simulink model "COV_sim_LQ_nonlin"  (R2023a)
settings: Solver=VariableStepAuto  StartTime=0.0  StopTime=tf  RelTol=1e-10
values from neighbouring files (symbols this model uses):
  alpha = 1/2.5    (= 0.4)    [COV_init_LQ_nonlin.m]
  c1 = feedback_pars(1)    [COV_init_LQ_nonlin.m]
  c2 = feedback_pars(2)    [COV_init_LQ_nonlin.m]
  c3 = feedback_pars(3)    [COV_init_LQ_nonlin.m]
  delta = 0.75    [COV_init_LQ_nonlin.m]
  dt = 0.1    [COV_init_LQ_nonlin.m]    (also in SLPIAHRD_transition.m = 0.02)
  ekf_sample_time = 0.02    [COV_init_LQ_nonlin.m]
  eta = 0.076    [COV_init_LQ_nonlin.m]
  h = 1/10    (= 0.1)    [COV_init_LQ_nonlin.m]    (also in mf_epid_ode_model_8comp.m = {})
  input_sample_time = 0.1    [COV_init_LQ_nonlin.m]
  k2 = 0.37    [COV_init_LQ_nonlin.m]
  k2_error = 1    [COV_init_LQ_nonlin.m]
  k3 = 0.1429    [COV_init_LQ_nonlin.m]
  k3_error = 1    [COV_init_LQ_nonlin.m]
  mu = 0.145    [COV_init_LQ_nonlin.m]
  N = numel(d_sim)-1    [Aggregator_B.m]    (also in Aggregator_C.m; COV_init_LQ_nonlin.m = 1; Main_MPC_Agent_v1.m = 168; Main_MPC_Agent_v2_Integral.m = P*Nr_Periods)
  p = 1/3    (= 0.333333333333)    [COV_init_LQ_nonlin.m]    (also in Main_MPC_Agent_v2_Integral.m = zeros(np,1); SLPIAHRD_transition.m = [1/2.5; 1/3; 1/3; 0.75; 0.6; 1/4; 1/4; 0.076; 1/10; 0.145])
  p_A = 1/4    (= 0.25)    [COV_init_LQ_nonlin.m]
  p_I = 1/4    (= 0.25)    [COV_init_LQ_nonlin.m]
  q = 0.6    [COV_init_LQ_nonlin.m]
  ref_sample_time = -1    [COV_init_LQ_nonlin.m]
  switchtime = 30    [COV_init_LQ_nonlin.m]
  u_max = k1    (= 0.5)    [COV_init_LQ_nonlin.m]
  u_min = 0    [COV_init_LQ_nonlin.m]
  x0 = [S0; L0; P0; A0; I0; R0; H0; D0]    [COV_init_LQ_nonlin.m]    (also in Main_MPC_Agent_v1.m = simx; Main_MPC_Agent_v2_Integral.m = simx; Main_MPC_Agent_v3.m = simx; Main_MPC_Agent_v5_Tp01.m = simx)
  z1_start = abs(x_ref(1, 2) - I0)    [COV_init_LQ_nonlin.m]
libraries: sharedTrackingLibrary x2
settings Model: PacingRate=0.001000  Creator=szeder  LastModifiedBy=ppolcz
settings SolverCC: ZeroCrossAlgorithm=Adaptive  AlgebraicLoopSolver=TrustRegion
settings OptimizationCC: ReuseModelBlockBuffer=off
settings DebuggingCC: UnconnectedInputMsg=warning  UnconnectedOutputMsg=warning  UnconnectedLineMsg=warning
settings ModelReferenceCC: EnableRefExpFcnMdlSchedulingChecks=on
settings RTWCC: DLArmComputeVersion=19.05

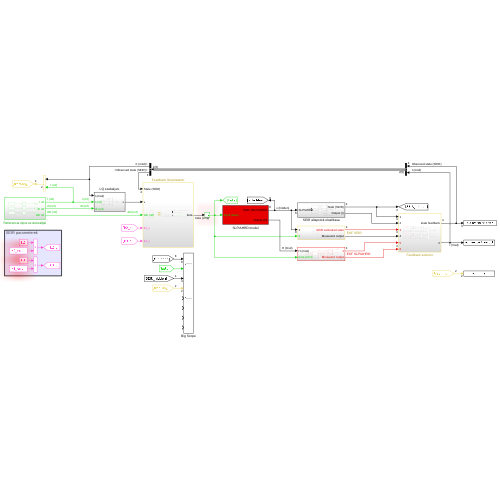
[thumbnail: Simulink's stored preview of the top-level diagram]
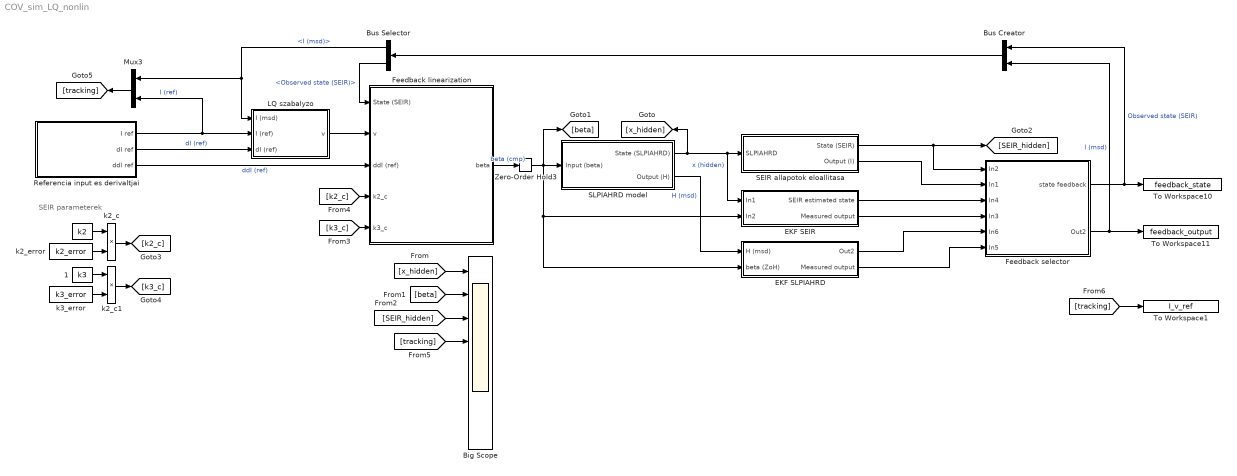
== system COV_sim_LQ_nonlin ==
  note: SEIR parameterek
  " " : Constant  Value=k2
  " 1" : Constant  Value=k3
  Big Scope : Scope  NumInputPorts=8
  Bus Creator : BusCreator  Inputs=2
  Bus Selector : BusSelector  OutputSignals=I (msd),Observed state (SEIR)
  EKF SEIR : Subsystem
  EKF SLPIAHRD : Subsystem
  Feedback linearization : Subsystem
  Feedback selector : Subsystem
  LQ szabalyzo : Subsystem
  Mux3 : Mux  Inputs=2
  Referencia input es derivaltjai : Subsystem
  SEIR allapotok eloallitasa : Subsystem
  SLPIAHRD model : Subsystem
  To Workspace1 : ToWorkspace  VariableName=I_v_ref  SaveFormat=Structure With Time  SampleTime=-1
  To Workspace10 : ToWorkspace  VariableName=feedback_state  SaveFormat=Timeseries  SampleTime=-1
  To Workspace11 : ToWorkspace  VariableName=feedback_output  SaveFormat=Timeseries  SampleTime=-1
  Zero-Order Hold3 : ZeroOrderHold  SampleTime=input_sample_time
  k2_c : Product
  k2_c1 : Product
  k2_error : Constant  Value=k2_error
  k3_error : Constant  Value=k3_error
  wires:
  Zero-Order Hold3/1 -> EKF SLPIAHRD/2(beta (ZoH)), EKF SEIR/2(In2), [beta], SLPIAHRD model/1(Input (beta))
  LQ szabalyzo/1(v) -> Feedback linearization/2(v)
  SLPIAHRD model/1(State (SLPIAHRD)) -> EKF SEIR/1(In1), SEIR allapotok eloallitasa/1(SLPIAHRD), [x_hidden]  "x (hidden)"
  SLPIAHRD model/2(Output (H)) -> EKF SLPIAHRD/1(H (msd))  "H (msd)"
  SEIR allapotok eloallitasa/1(State (SEIR)) -> [SEIR_hidden], Feedback selector/1(In2)
  Feedback selector/1(state feedback) -> To Workspace10/1, Bus Creator/1  "Observed state (SEIR)"
  Feedback selector/2(Out2) -> To Workspace11/1, Bus Creator/2  "I (msd)"
  SEIR allapotok eloallitasa/2(Output (I)) -> Feedback selector/2(In1)
  EKF SEIR/2(Measured output) -> Feedback selector/4(In3)
  EKF SEIR/1(SEIR estimated state) -> Feedback selector/3(In4)
  EKF SLPIAHRD/2(Measured output) -> Feedback selector/6(In5)
  EKF SLPIAHRD/1(Out2) -> Feedback selector/5(In6)
  Referencia input es derivaltjai/1(I ref) -> Mux3/2, LQ szabalyzo/2(I (ref))  "I (ref)"
  Referencia input es derivaltjai/2(dI ref) -> LQ szabalyzo/3(dI (ref))  "dI (ref)"
  Referencia input es derivaltjai/3(ddI ref) -> Feedback linearization/3(ddI (ref))  "ddI (ref)"
  [x_hidden] -> Big Scope/1
  [beta] -> Big Scope/2
  [SEIR_hidden] -> Big Scope/3
  " "/1 -> k2_c/1
  k2_error/1 -> k2_c/2
  [k2_c] -> Feedback linearization/4(k2_c)
  [k3_c] -> Feedback linearization/5(k3_c)
  k2_c/1 -> [k2_c]
  k2_c1/1 -> [k3_c]
  k3_error/1 -> k2_c1/2
  " 1"/1 -> k2_c1/1
  Mux3/1 -> [tracking]
  [tracking] -> Big Scope/4
  [tracking] -> To Workspace1/1
  Bus Creator/1 -> Bus Selector/1
  Bus Selector/1 -> Mux3/1, LQ szabalyzo/1(I (msd))  "<I (msd)>"
  Bus Selector/2 -> Feedback linearization/1(State (SEIR))  "<Observed state (SEIR)>"
  Feedback linearization/1(beta) -> Zero-Order Hold3/1  "beta (cmp)"

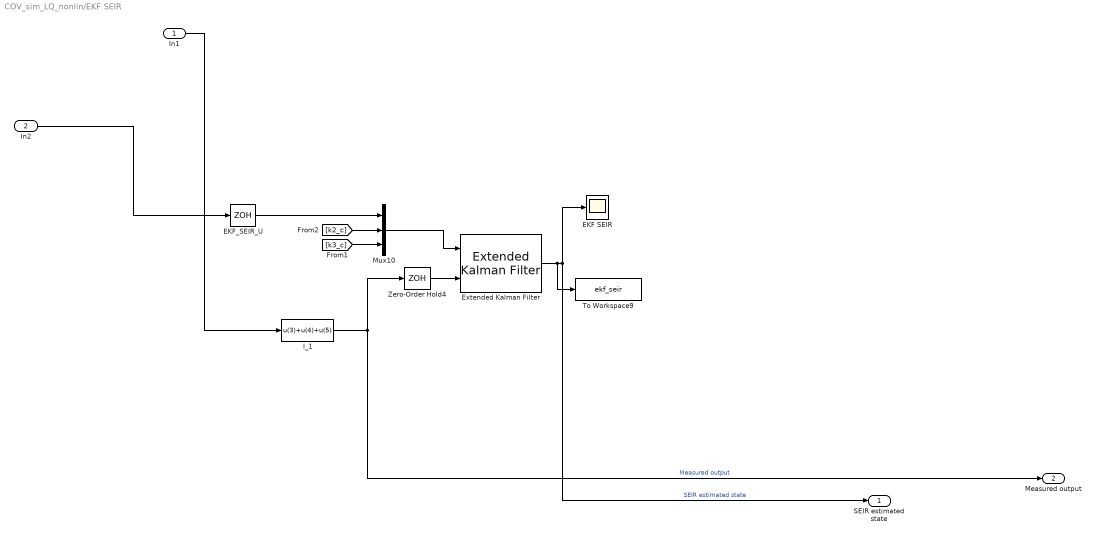
== system COV_sim_LQ_nonlin/EKF SEIR ==
  In1 : Inport
  In2 : Inport  Port=2
  EKF SEIR : Scope
  EKF_SEIR_U : ZeroOrderHold  SampleTime=ekf_sample_time
  Extended Kalman Filter : sharedTrackingLibrary/Extended Kalman Filter  StateTransitionFcn=SEIR_transition  HasStateTransitionJacobianFcn=off  HasAdditiveProcessNoise=Additive  ProcessNoise=ekf_seir_processcov  HasTimeVaryingProcessNoise=off  HasStateTransitionFcnExtraArgument=1  InitialState=ekf_seir_initialstate  InitialStateCovariance=ekf_seir_initcov  MeasurementFcn1=SEIR_measurement  HasMeasurementJacobianFcn1=off  HasMeasurementEnablePort1=off  HasAdditiveMeasurementNoise1=Additive  MeasurementNoise1=ekf_seir_measurecov  HasTimeVaryingMeasurementNoise1=off  HasMeasurementFcnExtraArgument1=0  HasMeasurementWrapping1=off  MeasurementFcn2=myMeasurementFcn  HasMeasurementJacobianFcn2=off  HasMeasurementEnablePort2=off  HasAdditiveMeasurementNoise2=Additive  MeasurementNoise2=1  HasTimeVaryingMeasurementNoise2=off  HasMeasurementFcnExtraArgument2=0  HasMeasurementWrapping2=off  MeasurementFcn3=myMeasurementFcn  HasMeasurementJacobianFcn3=off  HasMeasurementEnablePort3=off  HasAdditiveMeasurementNoise3=Additive  MeasurementNoise3=1  HasTimeVaryingMeasurementNoise3=off  HasMeasurementFcnExtraArgument3=0  HasMeasurementWrapping3=off  MeasurementFcn4=myMeasurementFcn  HasMeasurementJacobianFcn4=off  HasMeasurementEnablePort4=off  HasAdditiveMeasurementNoise4=Additive  MeasurementNoise4=1  HasTimeVaryingMeasurementNoise4=off  HasMeasurementFcnExtraArgument4=0  HasMeasurementWrapping4=off  MeasurementFcn5=myMeasurementFcn  HasMeasurementJacobianFcn5=off  HasMeasurementEnablePort5=off  HasAdditiveMeasurementNoise5=Additive  MeasurementNoise5=1  HasTimeVaryingMeasurementNoise5=off  HasMeasurementFcnExtraArgument5=0  HasMeasurementWrapping5=off  EnableMultirate=off  StateTransitionFcnSampleTime=1  MeasurementFcn1SampleTime=1  MeasurementFcn2SampleTime=1  MeasurementFcn3SampleTime=1  MeasurementFcn4SampleTime=1  MeasurementFcn5SampleTime=1  UseCurrentEstimator=on  OutputStateCovariance=off  DataType=double  SampleTime=ekf_sample_time  NumberOfMeasurements=1
  I_1 : MATLABFcn  MATLABFcn=u(3)+u(4)+u(5)  OutputDimensions=1  Output1D=off
  Mux10 : Mux  Inputs=3
  To Workspace9 : ToWorkspace  VariableName=ekf_seir  SaveFormat=Timeseries  SampleTime=-1
  Zero-Order Hold4 : ZeroOrderHold  SampleTime=ekf_sample_time
  SEIR estimated state : Outport
  Measured output : Outport  Port=2
  wires:
  EKF_SEIR_U/1 -> Mux10/1
  [k3_c] -> Mux10/3
  Zero-Order Hold4/1 -> Extended Kalman Filter/2
  In2/1 -> EKF_SEIR_U/1
  I_1/1 -> Measured output/1, Zero-Order Hold4/1  "Measured output"
  Mux10/1 -> Extended Kalman Filter/1
  Extended Kalman Filter/1 -> SEIR estimated state/1, EKF SEIR/1, To Workspace9/1  "SEIR estimated state"
  [k2_c] -> Mux10/2
  In1/1 -> I_1/1

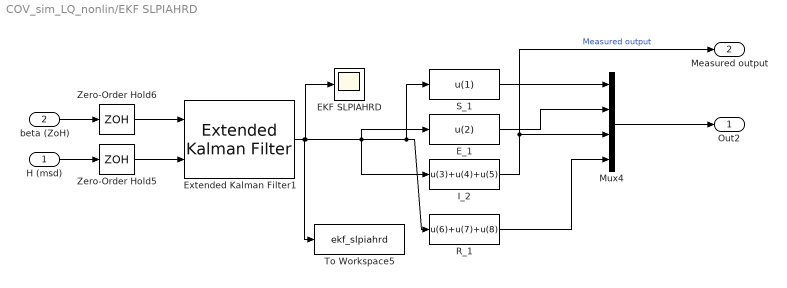
== system COV_sim_LQ_nonlin/EKF SLPIAHRD ==
  H (msd) : Inport
  beta (ZoH) : Inport  Port=2
  EKF SLPIAHRD : Scope
  E_1 : MATLABFcn  MATLABFcn=u(2)
  Extended Kalman Filter1 : sharedTrackingLibrary/Extended Kalman Filter  StateTransitionFcn=SLPIAHRD_transition  HasStateTransitionJacobianFcn=off  HasAdditiveProcessNoise=Additive  ProcessNoise=ekf_slpiahrd_processcov  HasTimeVaryingProcessNoise=off  HasStateTransitionFcnExtraArgument=1  InitialState=ekf_slpiahrd_initialstate  InitialStateCovariance=ekf_slpiahrd_initcov  MeasurementFcn1=SLPIAHRD_measurement  HasMeasurementJacobianFcn1=off  HasMeasurementEnablePort1=off  HasAdditiveMeasurementNoise1=Additive  MeasurementNoise1=ekf_slpiahrd_measurecov  HasTimeVaryingMeasurementNoise1=off  HasMeasurementFcnExtraArgument1=0  HasMeasurementWrapping1=off  MeasurementFcn2=myMeasurementFcn  HasMeasurementJacobianFcn2=off  HasMeasurementEnablePort2=off  HasAdditiveMeasurementNoise2=Additive  MeasurementNoise2=1  HasTimeVaryingMeasurementNoise2=off  HasMeasurementFcnExtraArgument2=0  HasMeasurementWrapping2=off  MeasurementFcn3=myMeasurementFcn  HasMeasurementJacobianFcn3=off  HasMeasurementEnablePort3=off  HasAdditiveMeasurementNoise3=Additive  MeasurementNoise3=1  HasTimeVaryingMeasurementNoise3=off  HasMeasurementFcnExtraArgument3=0  HasMeasurementWrapping3=off  MeasurementFcn4=myMeasurementFcn  HasMeasurementJacobianFcn4=off  HasMeasurementEnablePort4=off  HasAdditiveMeasurementNoise4=Additive  MeasurementNoise4=1  HasTimeVaryingMeasurementNoise4=off  HasMeasurementFcnExtraArgument4=0  HasMeasurementWrapping4=off  MeasurementFcn5=myMeasurementFcn  HasMeasurementJacobianFcn5=off  HasMeasurementEnablePort5=off  HasAdditiveMeasurementNoise5=Additive  MeasurementNoise5=1  HasTimeVaryingMeasurementNoise5=off  HasMeasurementFcnExtraArgument5=0  HasMeasurementWrapping5=off  EnableMultirate=off  StateTransitionFcnSampleTime=0.5  MeasurementFcn1SampleTime=0.5  MeasurementFcn2SampleTime=1  MeasurementFcn3SampleTime=1  MeasurementFcn4SampleTime=1  MeasurementFcn5SampleTime=1  UseCurrentEstimator=on  OutputStateCovariance=off  DataType=double  SampleTime=ekf_sample_time  NumberOfMeasurements=1
  I_2 : MATLABFcn  MATLABFcn=u(3)+u(4)+u(5)
  Mux4 : Mux
  R_1 : MATLABFcn  MATLABFcn=u(6)+u(7)+u(8)
  S_1 : MATLABFcn  MATLABFcn=u(1)
  To Workspace5 : ToWorkspace  VariableName=ekf_slpiahrd  SaveFormat=Timeseries  SampleTime=-1
  Zero-Order Hold5 : ZeroOrderHold  SampleTime=ekf_sample_time
  Zero-Order Hold6 : ZeroOrderHold  SampleTime=ekf_sample_time
  Out2 : Outport
  Measured output : Outport  Port=2
  wires:
  R_1/1 -> Mux4/4
  beta (ZoH)/1 -> Zero-Order Hold6/1
  S_1/1 -> Mux4/1
  Zero-Order Hold6/1 -> Extended Kalman Filter1/1
  E_1/1 -> Mux4/2
  Zero-Order Hold5/1 -> Extended Kalman Filter1/2
  Mux4/1 -> Out2/1
  Extended Kalman Filter1/1 -> S_1/1, R_1/1, E_1/1, I_2/1, EKF SLPIAHRD/1, To Workspace5/1
  H (msd)/1 -> Zero-Order Hold5/1
  I_2/1 -> Measured output/1, Mux4/3  "Measured output"

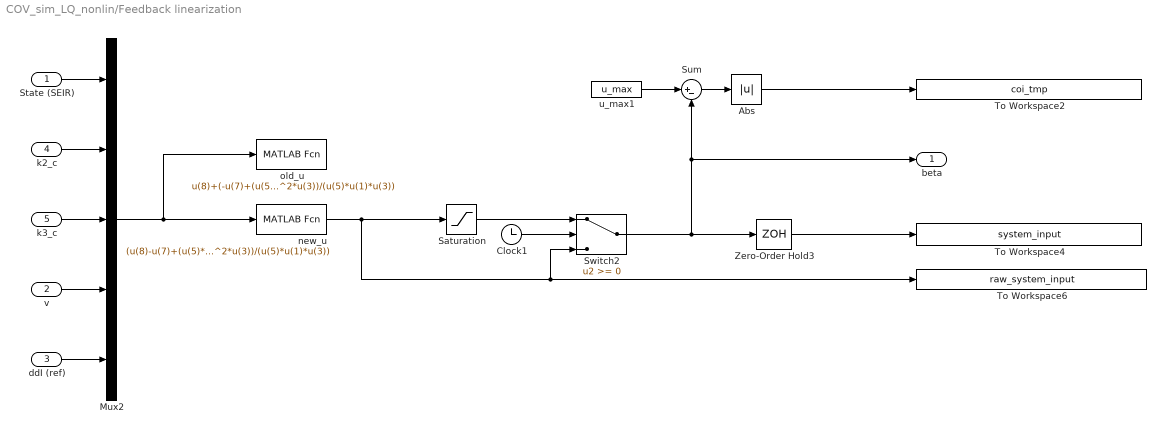
== system COV_sim_LQ_nonlin/Feedback linearization ==
  State (SEIR) : Inport
  v : Inport  Port=2
  ddI (ref) : Inport  Port=3
  k2_c : Inport  Port=4
  k3_c : Inport  Port=5
  " u_max1" : Constant  Value=u_max
  Abs : Abs  SaturateOnIntegerOverflow=off
  Clock1 : Clock
  Mux2 : Mux  Inputs=5
  Saturation : Saturate  UpperLimit=u_max  LowerLimit=u_min
  Sum : Sum  Inputs=|+-
  Switch2 : Switch  SaturateOnIntegerOverflow=off  InputSameDT=off
  To Workspace2 : ToWorkspace  VariableName=coi_tmp  SaveFormat=Timeseries  SampleTime=-1
  To Workspace4 : ToWorkspace  VariableName=system_input  SaveFormat=Timeseries  SampleTime=-1
  To Workspace6 : ToWorkspace  VariableName=raw_system_input  SaveFormat=Timeseries  SampleTime=-1
  Zero-Order Hold3 : ZeroOrderHold  SampleTime=input_sample_time
  new_u : MATLABFcn  MATLABFcn=(u(8)-u(7)+(u(5)*u(6)+u(5)^2)*u(2)-u(6)^2*u(3))/(u(5)*u(1)*u(3))
  old_u : MATLABFcn  MATLABFcn=u(8)+(-u(7)+(u(5)*u(6)+u(5)^2)*u(2)-u(6)^2*u(3))/(u(5)*u(1)*u(3))
  beta : Outport
  wires:
  State (SEIR)/1 -> Mux2/1
  k3_c/1 -> Mux2/3
  Zero-Order Hold3/1 -> To Workspace4/1
  k2_c/1 -> Mux2/2
  Mux2/1 -> new_u/1, old_u/1
  ddI (ref)/1 -> Mux2/5
  Clock1/1 -> Switch2/2
  Switch2/1 -> Sum/2, beta/1, Zero-Order Hold3/1
  new_u/1 -> Saturation/1, Switch2/3, To Workspace6/1
  v/1 -> Mux2/4
  Saturation/1 -> Switch2/1
  " u_max1"/1 -> Sum/1
  Sum/1 -> Abs/1
  Abs/1 -> To Workspace2/1

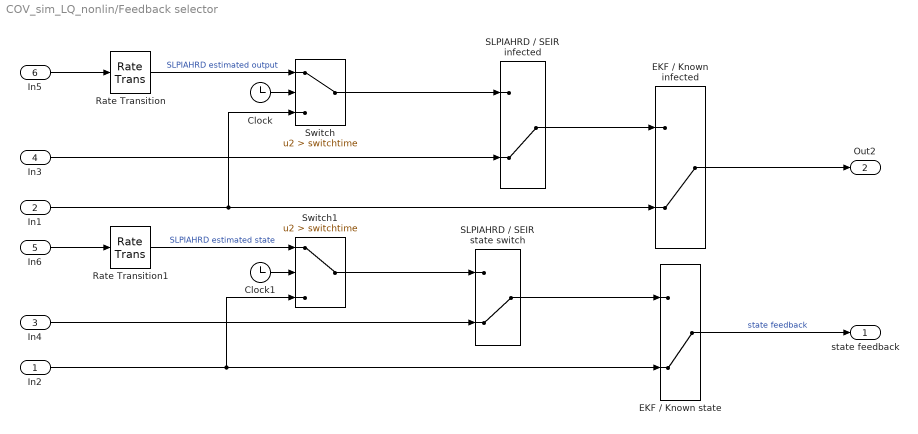
== system COV_sim_LQ_nonlin/Feedback selector ==
  In2 : Inport
  In1 : Inport  Port=2
  In4 : Inport  Port=3
  In3 : Inport  Port=4
  In6 : Inport  Port=5
  In5 : Inport  Port=6
  Clock : Clock
  Clock1 : Clock
  EKF / Known infected : ManualSwitch  CurrentSetting=0
  EKF / Known state : ManualSwitch  CurrentSetting=0
  Rate Transition : RateTransition  Integrity=off  OutPortSampleTimeMultiple=2  OutPortSampleTime=ratetrans_sample_time
  Rate Transition1 : RateTransition  Integrity=off  OutPortSampleTime=ratetrans_sample_time
  SLPIAHRD / SEIR infected : ManualSwitch  CurrentSetting=0
  SLPIAHRD / SEIR state switch : ManualSwitch  CurrentSetting=0
  Switch : Switch  Criteria=u2 > Threshold  Threshold=switchtime  SaturateOnIntegerOverflow=off  InputSameDT=off
  Switch1 : Switch  Criteria=u2 > Threshold  Threshold=switchtime  SaturateOnIntegerOverflow=off  InputSameDT=off
  state feedback : Outport
  Out2 : Outport  Port=2
  wires:
  Switch1/1 -> SLPIAHRD / SEIR state switch/1
  In4/1 -> SLPIAHRD / SEIR state switch/2
  In3/1 -> SLPIAHRD / SEIR infected/2
  Rate Transition1/1 -> Switch1/1  "SLPIAHRD estimated state"
  EKF / Known infected/1 -> Out2/1
  Clock/1 -> Switch/2
  In5/1 -> Rate Transition/1
  Rate Transition/1 -> Switch/1  "SLPIAHRD estimated output"
  In6/1 -> Rate Transition1/1
  EKF / Known state/1 -> state feedback/1  "state feedback"
  In1/1 -> Switch/3, EKF / Known infected/2
  In2/1 -> EKF / Known state/2, Switch1/3
  Switch/1 -> SLPIAHRD / SEIR infected/1
  SLPIAHRD / SEIR infected/1 -> EKF / Known infected/1
  SLPIAHRD / SEIR state switch/1 -> EKF / Known state/1
  Clock1/1 -> Switch1/2

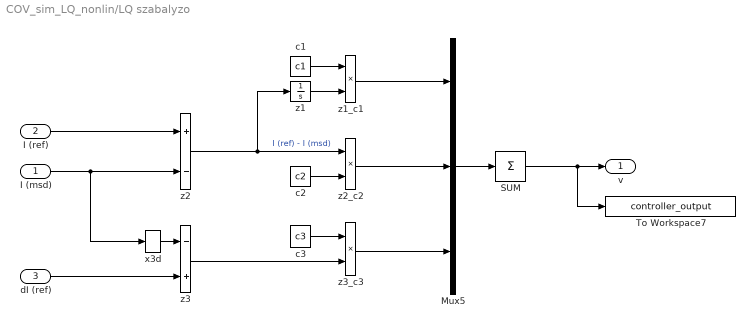
== system COV_sim_LQ_nonlin/LQ szabalyzo ==
  I (msd) : Inport
  I (ref) : Inport  Port=2
  dI (ref) : Inport  Port=3
  " c1" : Constant  Value=c1
  " c2" : Constant  Value=c2
  " c3" : Constant  Value=c3
  Mux5 : Mux  Inputs=3
  SUM : Sum  Inputs=+
  To Workspace7 : ToWorkspace  VariableName=controller_output  SaveFormat=Timeseries  SampleTime=-1
  x3d : Derivative
  z1 : Integrator  InitialCondition=z1_start
  z1_c1 : Product
  z2 : Sum  Inputs=+-
  z2_c2 : Product
  z3 : Sum  Inputs=-+
  z3_c3 : Product
  v : Outport
  wires:
  Mux5/1 -> SUM/1
  dI (ref)/1 -> z3/2
  " c1"/1 -> z1_c1/1
  I (msd)/1 -> x3d/1, z2/2
  z3_c3/1 -> Mux5/3
  z2_c2/1 -> Mux5/2
  SUM/1 -> v/1, To Workspace7/1
  x3d/1 -> z3/1
  " c2"/1 -> z2_c2/2
  I (ref)/1 -> z2/1
  z3/1 -> z3_c3/2
  z2/1 -> z2_c2/1, z1/1  "I (ref) - I (msd)"
  z1/1 -> z1_c1/2
  z1_c1/1 -> Mux5/1
  " c3"/1 -> z3_c3/1

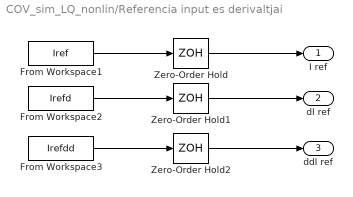
== system COV_sim_LQ_nonlin/Referencia input es derivaltjai ==
  From Workspace1 : FromWorkspace  VariableName=Iref  SampleTime=dt
  From Workspace2 : FromWorkspace  VariableName=Irefd  SampleTime=dt
  From Workspace3 : FromWorkspace  VariableName=Irefdd  SampleTime=dt
  Zero-Order Hold : ZeroOrderHold  SampleTime=ref_sample_time
  Zero-Order Hold1 : ZeroOrderHold  SampleTime=ref_sample_time
  Zero-Order Hold2 : ZeroOrderHold  SampleTime=ref_sample_time
  I ref : Outport
  dI ref : Outport  Port=2
  ddI ref : Outport  Port=3
  wires:
  From Workspace1/1 -> Zero-Order Hold/1
  Zero-Order Hold2/1 -> ddI ref/1
  From Workspace3/1 -> Zero-Order Hold2/1
  From Workspace2/1 -> Zero-Order Hold1/1
  Zero-Order Hold1/1 -> dI ref/1
  Zero-Order Hold/1 -> I ref/1

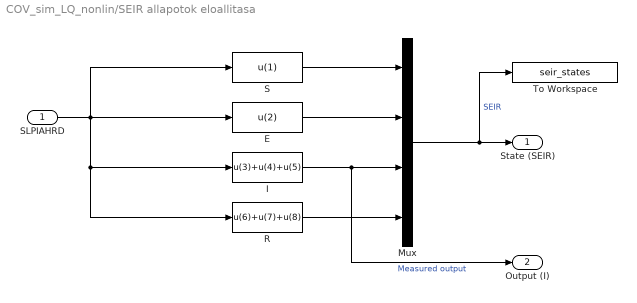
== system COV_sim_LQ_nonlin/SEIR allapotok eloallitasa ==
  SLPIAHRD : Inport
  E : MATLABFcn  MATLABFcn=u(2)
  I : MATLABFcn  MATLABFcn=u(3)+u(4)+u(5)
  Mux : Mux
  R : MATLABFcn  MATLABFcn=u(6)+u(7)+u(8)
  S : MATLABFcn  MATLABFcn=u(1)
  To Workspace : ToWorkspace  VariableName=seir_states  SaveFormat=Structure With Time  SampleTime=-1
  State (SEIR) : Outport
  Output (I) : Outport  Port=2
  wires:
  R/1 -> Mux/4
  S/1 -> Mux/1
  E/1 -> Mux/2
  Mux/1 -> To Workspace/1, State (SEIR)/1  "SEIR"
  I/1 -> Output (I)/1, Mux/3  "Measured output"
  SLPIAHRD/1 -> S/1, R/1, I/1, E/1

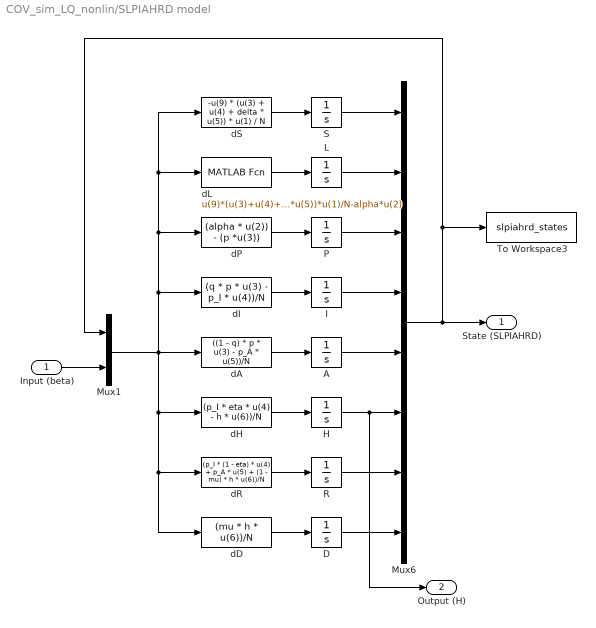
== system COV_sim_LQ_nonlin/SLPIAHRD model ==
  Input (beta) : Inport
  A : Integrator  InitialCondition=x0(5)
  D : Integrator  InitialCondition=x0(8)
  H : Integrator  InitialCondition=x0(6)
  I : Integrator  InitialCondition=x0(4)
  L : Integrator  InitialCondition=x0(2)
  Mux1 : Mux  Inputs=2
  Mux6 : Mux  Inputs=8
  P : Integrator  InitialCondition=x0(3)
  R : Integrator  InitialCondition=x0(7)
  S : Integrator  InitialCondition=x0(1)
  To Workspace3 : ToWorkspace  VariableName=slpiahrd_states  SaveFormat=Timeseries  SampleTime=-1
  dA : MATLABFcn  MATLABFcn=((1 - q) * p * u(3) - p_A * u(5))/N  Output1D=off
  dD : MATLABFcn  MATLABFcn=(mu * h * u(6))/N  Output1D=off
  dH : MATLABFcn  MATLABFcn=(p_I * eta * u(4) - h * u(6))/N  Output1D=off
  dI : MATLABFcn  MATLABFcn=(q * p * u(3) - p_I * u(4))/N  Output1D=off
  dL : MATLABFcn  MATLABFcn=u(9)*(u(3)+u(4)+delta*u(5))*u(1)/N-alpha*u(2)  Output1D=off
  dP : MATLABFcn  MATLABFcn=(alpha * u(2)) - (p *u(3))  Output1D=off
  dR : MATLABFcn  MATLABFcn=(p_I * (1 - eta) * u(4) + p_A * u(5) + (1 - mu) * h * u(6))/N  Output1D=off
  dS : MATLABFcn  MATLABFcn=-u(9) * (u(3) + u(4) + delta * u(5)) * u(1) / N  Output1D=off
  State (SLPIAHRD) : Outport
  Output (H) : Outport  Port=2
  wires:
  R/1 -> Mux6/7
  dL/1 -> L/1
  S/1 -> Mux6/1
  D/1 -> Mux6/8
  dH/1 -> H/1
  dA/1 -> A/1
  Input (beta)/1 -> Mux1/2
  Mux6/1 -> To Workspace3/1, Mux1/1, State (SLPIAHRD)/1
  L/1 -> Mux6/2
  dP/1 -> P/1
  dI/1 -> I/1
  Mux1/1 -> dP/1, dL/1, dS/1, dI/1, dR/1, dD/1, dH/1, dA/1
  dS/1 -> S/1
  I/1 -> Mux6/4
  dR/1 -> R/1
  A/1 -> Mux6/5
  dD/1 -> D/1
  P/1 -> Mux6/3
  H/1 -> Output (H)/1, Mux6/6
